simulink model "prodinvsys_sim_ol"  (R2021b)
settings: Solver=ode15s  StartTime=0.0  StopTime=250  RelTol=1e-3  AbsTol=1e-6
values from neighbouring files (symbols this model uses):
  thetap1 = 3    [run_sim_ol.m]
  thetap2 = 1    [run_sim_ol.m]
  Ts = 1    [run_sim_ol.m]    (also in test_prod_inv_sys_dt.m)
undefined symbols (not defined in the file or in its folder): DiscIntNeverNeededParam
settings Model: Creator=derivera  LastModifiedBy=billtubbs
settings SolverCC: AutoScaleAbsTol=off  AlgebraicLoopSolver=TrustRegion
settings DataIOCC: SaveFormat=Array  SignalLoggingSaveFormat=ModelDataLogs  ReturnWorkspaceOutputs=off
settings OptimizationCC: BooleanDataType=off  LifeSpan=inf
settings DebuggingCC: SaveWithParameterizedLinksMsg=none  UnderspecifiedInitializationDetection=Classic  MergeDetectMultiDrivingBlocksExec=none  SignalResolutionControl=TryResolveAllWithWarning  MultiTaskDSMMsg=warning  MultiTaskCondExecSysMsg=none  SFUnexpectedBacktrackingDiag=warning  SFNoUnconditionalDefaultTransitionDiag=warning  SFExecutionAtInitializationDiag=none  SFMachineParentedDataDiag=warning  ArithmeticOperatorsInVariantConditions=warning
settings HardwareCC: ProdBitPerPointer=32  ProdBitPerSizeT=32  ProdBitPerPtrDiffT=32  ProdLargestAtomicFloat=None  ProdIntDivRoundTo=Undefined  ProdEndianess=Unspecified  ProdWordSize=32  ProdHWDeviceType=32-bit Generic  TargetUnknown=on
settings ModelReferenceCC: PropagateSignalLabelsOutOfModel=off
settings SFSimCC: SimUseLocalCustomCode=off  CustomCodeUndefinedFunction=UseInterfaceOnly
settings RTWCC: RTWUseLocalCustomCode=off
settings CodeAppCC: StateflowObjectComments=on
settings GRTTargetCC: TargetLangStandard=C89/C90 (ANSI)  CombineOutputUpdateFcns=off  GRTInterface=on
settings ConfigComp: CovMetricSettings=dw  CovSaveCumulativeToWorkspaceVar=on  CovSaveSingleToWorkspaceVar=on  CovExternalEMLEnable=off  CovSFcnEnable=off

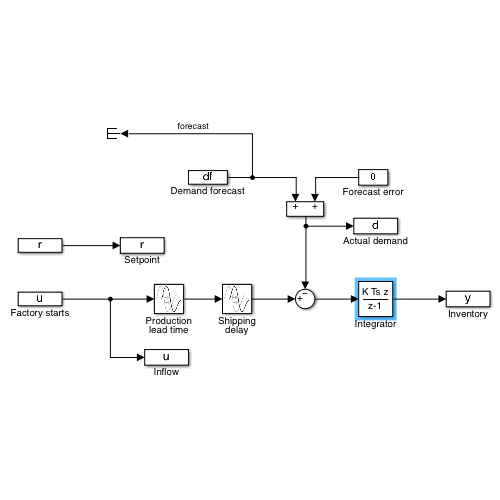
[thumbnail: Simulink's stored preview of the top-level diagram]
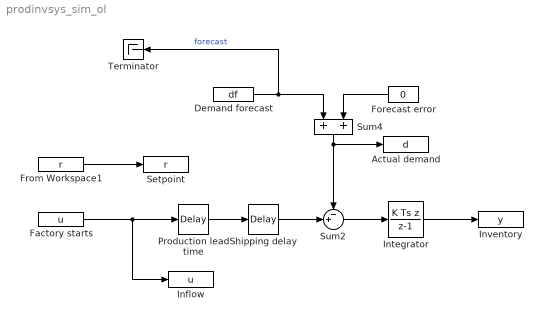
== system prodinvsys_sim_ol ==
  Actual demand : ToWorkspace  VariableName=d  SampleTime=Ts
  Demand forecast : FromWorkspace  VariableName=df
  Factory starts : FromWorkspace  VariableName=u
  Forecast error : Constant  Value=0
  From Workspace1 : FromWorkspace  VariableName=r
  Inflow : ToWorkspace  VariableName=u  SampleTime=Ts
  Integrator : DiscreteIntegrator  IntegratorMethod=Integration: Backward Euler  gainval=1  SampleTime=-1  ICPrevOutput=DiscIntNeverNeededParam  ICPrevScaledInput=DiscIntNeverNeededParam
  Inventory : ToWorkspace  VariableName=y  SampleTime=Ts
  Production lead time : TransportDelay  DelayTime=thetap1
  Setpoint : ToWorkspace  VariableName=r  SampleTime=Ts
  Shipping delay : TransportDelay  DelayTime=thetap2
  Sum2 : Sum  Inputs=-+|
  Sum4 : Sum  InputSameDT=on  SaturateOnIntegerOverflow=on  OutDataTypeStr=Inherit: Same as first input
  Terminator : Terminator
  wires:
  Sum4/1 -> Sum2/1, Actual demand/1
  Factory starts/1 -> Production lead time/1, Inflow/1
  Demand forecast/1 -> Sum4/1, Terminator/1  "forecast"
  Forecast error/1 -> Sum4/2
  Integrator/1 -> Inventory/1
  Sum2/1 -> Integrator/1
  From Workspace1/1 -> Setpoint/1
  Production lead time/1 -> Shipping delay/1
  Shipping delay/1 -> Sum2/2
